simulink model "Priority vs Plain Ticket Gate"  (R2018a)
settings: Solver=VariableStepAuto  StartTime=0.0  StopTime=100  RelTol=1e-3
undefined symbols (not defined in the file): m, n
settings Model: Creator=user  LastModifiedBy=user

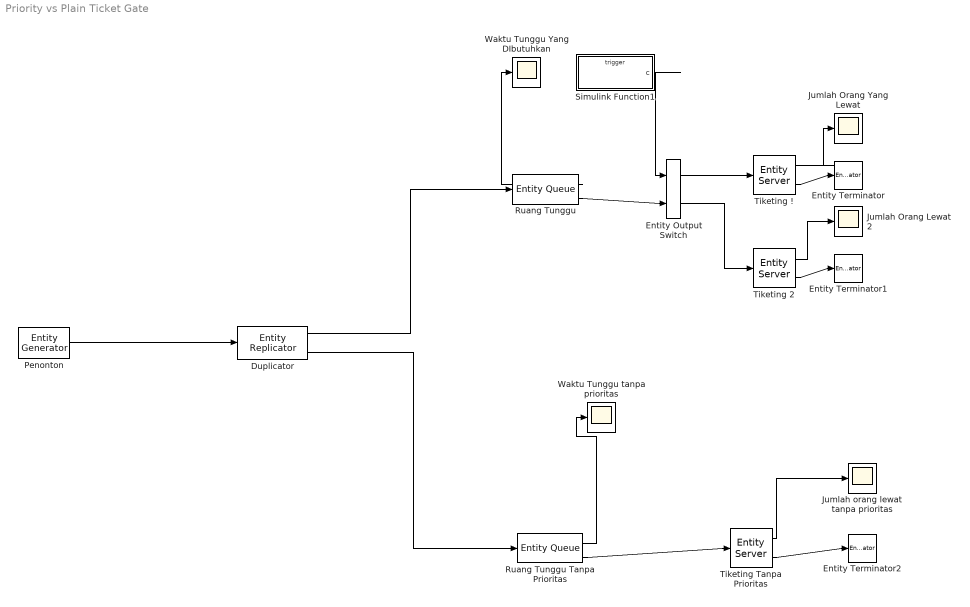
== system Priority vs Plain Ticket Gate ==
  Duplicator : EntityReplicator  InputPortMessageModes=m  OutputPortMessageModes=m,m
  Entity Output Switch : EntityOutputSwitch  InputPortMessageModes=m,m  OutputPortMessageModes=m,m  SwitchingCriterion=From control port  SwitchAttributeName=Attribute1  InitialPortSelection=2
      settings: InputPortMap=u0,u1
  Entity Terminator : EntityTerminator  InputPortMessageModes=m
  Entity Terminator1 : EntityTerminator  InputPortMessageModes=m
  Entity Terminator2 : EntityTerminator  InputPortMessageModes=m
  Jumlah Orang Lewat 2 : Scope
  Jumlah Orang Yang Lewat : Scope
  Jumlah orang lewat tanpa prioritas : Scope
  Penonton : EntityGenerator  OutputPortMessageModes=m  TimeSource=MATLAB action  IntergenerationTimeAction=|  GenerateAction=entity.Class = randi([1 3]);  AttributeName=Class  AttributeInitialValue=0  EntityType=Structured  EntityTypeName=Penonton
      | mean = 0.5;
      | dt = mean*rand();
  Ruang Tunggu : EntityQueue  InputPortMessageModes=m  OutputPortMessageModes=n,m  Capacity=inf  PrioritySource=Class  SortingDirection=Descending  ExitAction=|  AverageWait=on
      | if entity.Class == 1 
      |     SwitchCtrl(1);
      | else 
      |     SwitchCtrl(2);
      | end
      settings: OutputPortMap=o2,o5
  Ruang Tunggu Tanpa Prioritas : EntityQueue  InputPortMessageModes=m  OutputPortMessageModes=n,m  Capacity=inf  PrioritySource=Class  SortingDirection=Descending  AverageWait=on
      settings: OutputPortMap=o2,o5
  Simulink Function1 : Subsystem  TreatAsAtomicUnit=on
  Tiketing ! : EntityServer  InputPortMessageModes=m  OutputPortMessageModes=n,m  ServiceTimeValue=1  EntryAction=|  NumberEntitiesDeparted=on
      | persistent nEntered
      | if isempty(nEntered)
      |     nEntered = 0;
      | end
      | 
      | 
      |        
      | nEntered = nEntered + 1;
      settings: OutputPortMap=o0,o9
  Tiketing 2 : EntityServer  InputPortMessageModes=m  OutputPortMessageModes=n,m  ServiceTimeValue=1  EntryAction=|  NumberEntitiesDeparted=on
      | persistent nEntered
      | if isempty(nEntered)
      |     nEntered = 0;
      | end
      | 
      | 
      |        
      | nEntered = nEntered + 1;
      settings: OutputPortMap=o0,o9
  Tiketing Tanpa Prioritas : EntityServer  InputPortMessageModes=m  OutputPortMessageModes=n,m  ServiceTimeValue=1  NumberEntitiesDeparted=on
      settings: OutputPortMap=o0,o9
  Waktu Tunggu Yang DIbutuhkan : Scope
  Waktu Tunggu tanpa prioritas : Scope
  wires:
  Penonton/1 -> Duplicator/1
  Ruang Tunggu/2 -> Entity Output Switch/2
  Simulink Function1/1(c) -> Entity Output Switch/1
  Entity Output Switch/1 -> Tiketing !/1
  Tiketing !/2 -> Entity Terminator/1
  Tiketing !/1 -> Jumlah Orang Yang Lewat/1
  Entity Output Switch/2 -> Tiketing 2/1
  Tiketing 2/1 -> Jumlah Orang Lewat 2/1
  Tiketing 2/2 -> Entity Terminator1/1
  Ruang Tunggu/1 -> Waktu Tunggu Yang DIbutuhkan/1
  Ruang Tunggu Tanpa Prioritas/1 -> Waktu Tunggu tanpa prioritas/1
  Duplicator/2 -> Ruang Tunggu Tanpa Prioritas/1
  Tiketing Tanpa Prioritas/2 -> Entity Terminator2/1
  Ruang Tunggu Tanpa Prioritas/2 -> Tiketing Tanpa Prioritas/1
  Tiketing Tanpa Prioritas/1 -> Jumlah orang lewat tanpa prioritas/1
  Duplicator/1 -> Ruang Tunggu/1

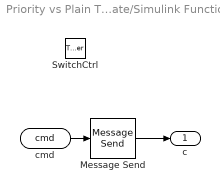
== system Priority vs Plain Ticket Gate/Simulink Function1 ==
  SwitchCtrl : TriggerPort  TriggerType=function-call  IsSimulinkFunction=on  FunctionName=SwitchCtrl  VariantControl=Variant
  Message Send : MessageSend  OutputPortMessageModes=m
      settings: InputPortMap=u1
  cmd : ArgIn  ArgumentName=cmd
  c : Outport
  wires:
  cmd/1 -> Message Send/1
  Message Send/1 -> c/1
